simulink model "tank_simulator"  (R2023b)
settings: Solver=VariableStepAuto  StartTime=0.0  StopTime=simtime  RelTol=1e-3
values from neighbouring files (symbols this model uses):
  initial_state = ((maxinitialstate-mininitialstate).*rand(param.nx,1) + mininitialstate)/10    [main_data_generator.m]    (also in main_simulink_3tanks.m = (maxinitialstate-mininitialstate).*rand(param.nx,1) + minini)
undefined symbols (not defined in the file or in its folder): param
libraries: simulink x1, dspsrcs4 x1
settings Model: Creator=danilo  LastModifiedBy=danilo

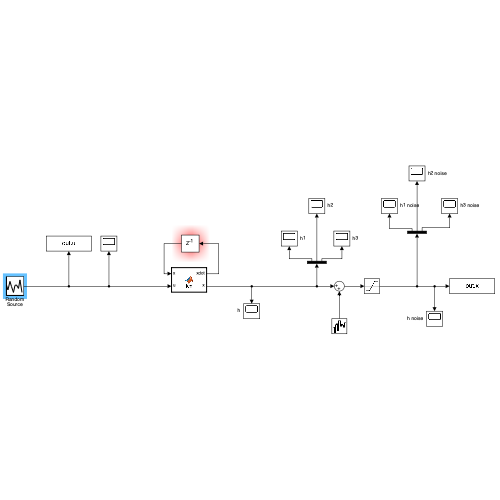
[thumbnail: Simulink's stored preview of the top-level diagram]
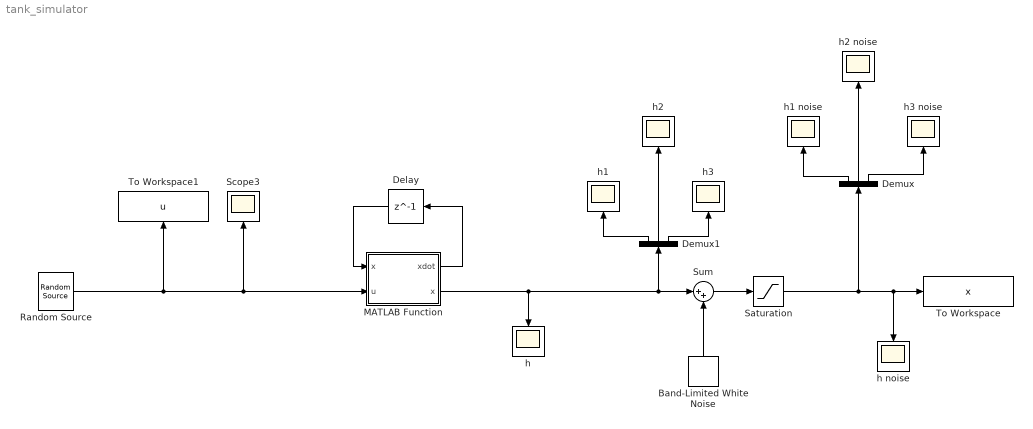
== system tank_simulator ==
  Band-Limited White Noise : simulink/Sources/Band-Limited White Noise  Cov=param.noisePower  Ts=param.Ts  seed=[23341]
  Delay : Delay  DelayLength=1  InitialCondition=initial_state  SampleTime=param.Ts
  Demux : Demux  Outputs=3
  Demux1 : Demux  Outputs=3
  MATLAB Function : MATLAB Function  TreatAsAtomicUnit=on
  Random Source : dspsrcs4/Random Source  SrcType=Uniform  NormMethod=Ziggurat  CltLength=12  MinVal=10  MaxVal=100  MeanVal=0  VarVal=1  RepMode=Not repeatable  rawSeed=2  IsInherit=off  SampMode=Discrete  SampTime=4  SampFrame=1  DataType=Double  OutComplex=Real  OutputFrames=off
  Saturation : Saturate  UpperLimit=inf  LowerLimit=0
  Scope3 : Scope
  Sum : Sum  Inputs=|++
  To Workspace : ToWorkspace  VariableName=x  SampleTime=param.Ts
  To Workspace1 : ToWorkspace  VariableName=u  SampleTime=param.Ts
  h{,1..3} (4 alike) : Scope
  h noise : Scope
  h1 noise : Scope
  h2 noise : Scope
  h3 noise : Scope
  wires:
  Random Source/1 -> MATLAB Function/2(u), Scope3/1, To Workspace1/1
  MATLAB Function/1(xdot) -> Delay/1
  Delay/1 -> MATLAB Function/1("x ")
  Demux/1 -> h1 noise/1
  Demux/2 -> h2 noise/1
  Demux/3 -> h3 noise/1
  Sum/1 -> Saturation/1
  Band-Limited White Noise/1 -> Sum/2
  Demux1/2 -> h2/1
  Demux1/1 -> h1/1
  Demux1/3 -> h3/1
  Saturation/1 -> To Workspace/1, h noise/1, Demux/1
  MATLAB Function/2(x) -> Demux1/1, Sum/1, h/1

== matlab function tank_simulator/MATLAB Function ==
  data: x input; u input; xdot output; x output; param parameter
 function [xdot,x]= fcn(x,u,param)


if x(1)>=0
    radx1 = sqrt(2*param.g*x(1));
else
    radx1 = 0;
end
if x(2)>=0
    radx2 = sqrt(2*param.g*x(2));
else
    radx2 = 0;
end
if x(3)>=0
    radx3 = sqrt(2*param.g*x(3));
else
    radx3 = 0;
end
xdot = zeros(3,1);

xdot(1) = x(1) + param.Ts*(-param.a1/param.A1*radx1+param.k1*param.a3/param.A1*radx3+param.ku*u(1)/param.A1);    
xdot(2) = x(2) + param.Ts*(-param.a2/param.A2*radx2+param.k2*param.a1/param.A2*radx1);        
xdot(3) = x(3) + param.Ts*(-param.a3/param.A3*radx3+param.k3*param.a2/param.A3*radx2);
